simulink model "simulink_non_lineare"  (R2025b)
settings: Solver=ode45  StartTime=0.0  StopTime=2  MaxStep=1e-6  RelTol=1e-3
values from neighbouring files (symbols this model uses):
  k1 = 0.10    (= 0.1)    [main.m]
  k2 = 1.50    (= 1.5)    [main.m]
  k3 = 0.12    [main.m]
  k4 = 2.50    (= 2.5)    [main.m]
  ue = (k1 * sqrt(x1e)) / k4    [main.m]
  x1e = a1_eq    (= 0.0235)    [main.m]
  x2e = a2_eq    (= 3.67)    [main.m]
libraries: cstblocks x1
settings Model: Creator=porpo  LastModifiedBy=porpo

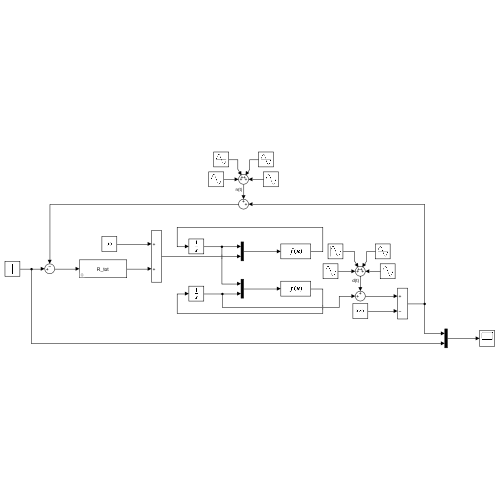
[thumbnail: Simulink's stored preview of the top-level diagram]
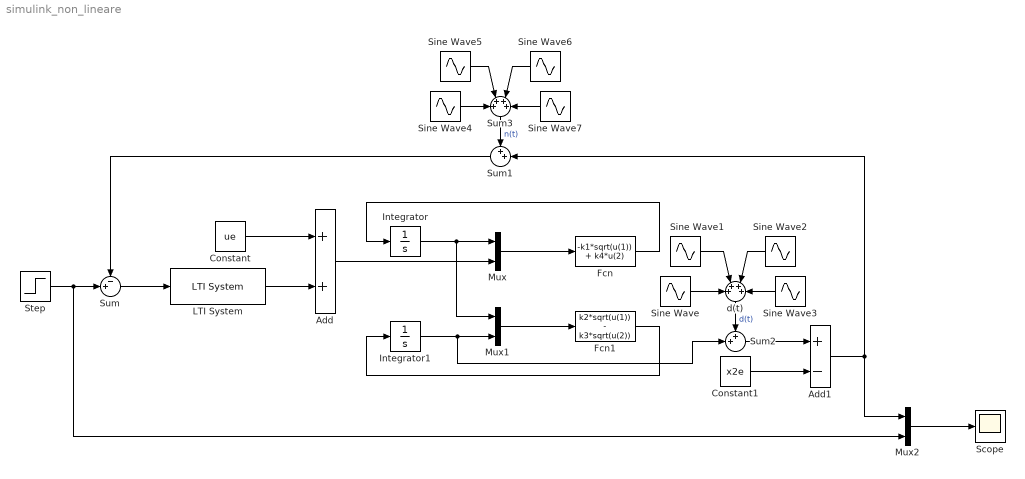
== system simulink_non_lineare ==
  Add : Sum
  Add1 : Sum  Inputs=+-
  Constant : Constant  Value=ue
  Constant1 : Constant  Value=x2e
  Fcn : Fcn  Expr=-k1*sqrt(u(1)) + k4*u(2)
  Fcn1 : Fcn  Expr=k2*sqrt(u(1)) - k3*sqrt(u(2))
  Integrator : Integrator  InitialCondition=x1e  LowerSaturationLimit=0
  Integrator1 : Integrator  InitialCondition=x2e  LowerSaturationLimit=0
  LTI System : cstblocks/LTI System  sys=R_tot  IC=[]  PadeOrder=0
  Mux : Mux  Inputs=2
  Mux1 : Mux  Inputs=2
  Mux2 : Mux  Inputs=2
  Scope : Scope
      settings: ActiveDisplayYMinimum=-11.251007967273763  ActiveDisplayYMaximum=101.25907170546388
  Sine Wave : Sin  Frequency=0.1  SampleTime=0
  Sine Wave1 : Sin  Frequency=0.2  SampleTime=0
  Sine Wave2 : Sin  Frequency=0.3  SampleTime=0
  Sine Wave3 : Sin  Frequency=0.4  SampleTime=0
  Sine Wave4 : Sin  Amplitude=2.5  Frequency=1e5*1  SampleTime=0
  Sine Wave5 : Sin  Amplitude=2.5  Frequency=1e5*2  SampleTime=0
  Sine Wave6 : Sin  Amplitude=2.5  Frequency=1e5*3  SampleTime=0
  Sine Wave7 : Sin  Amplitude=2.5  Frequency=1e5*4  SampleTime=0
  Step : Step  Time=0  After=50  SampleTime=0
  Sum : Sum  Inputs=-+|
  Sum1 : Sum  Inputs=++|
  Sum2 : Sum  Inputs=++|
  Sum3 : Sum  Inputs=++++
  d(t) : Sum  Inputs=++++
  wires:
  Integrator/1 -> Mux1/1, Mux/1
  Mux/1 -> Fcn/1
  Fcn/1 -> Integrator/1
  Integrator1/1 -> Sum2/2, Mux1/2
  Mux1/1 -> Fcn1/1
  Fcn1/1 -> Integrator1/1
  Constant/1 -> Add/1
  LTI System/1 -> Add/2
  Add/1 -> Mux/2
  Constant1/1 -> Add1/2
  Sum/1 -> LTI System/1
  Step/1 -> Mux2/2, Sum/2
  Add1/1 -> Sum1/2, Mux2/1
  Mux2/1 -> Scope/1
  Sum2/1 -> Add1/1
  d(t)/1 -> Sum2/1  "d(t)"
  Sine Wave/1 -> d(t)/1
  Sine Wave1/1 -> d(t)/2
  Sine Wave2/1 -> d(t)/3
  Sine Wave3/1 -> d(t)/4
  Sum1/1 -> Sum/1
  Sum3/1 -> Sum1/1  "n(t)"
  Sine Wave7/1 -> Sum3/4
  Sine Wave6/1 -> Sum3/3
  Sine Wave5/1 -> Sum3/2
  Sine Wave4/1 -> Sum3/1
